simulink model "MJrlsfiltersystemidentification"  (R2023a)
settings: Solver=FixedStepDiscrete  StartTime=0.0  StopTime=Inf  RelTol=1e-3  EnableMultiTasking=on
PreLoadFcn:
  | Ts = 1/1e4;
  | L = 1024;
libraries: dspsrcs4 x2, dspsnks4 x1, dspmathops x1, dspadpt3 x1
CloseFcn:
  | clear Ts L
  | close all force
settings Model: Creator=The MathWorks, Inc.  LastModifiedBy=janssonm
settings SolverCC: AlgebraicLoopSolver=TrustRegion  MaxZcPerStep=1
settings DataIOCC: LimitDataPoints=on  SaveFormat=Array  ReturnWorkspaceOutputs=off
settings OptimizationCC: ReuseModelBlockBuffer=off  LifeSpan=inf  SimCompilerOptimization=on
settings DebuggingCC: UnderspecifiedInitializationDetection=Classic  MergeDetectMultiDrivingBlocksExec=none  SolverPrmCheckMsg=warning  UnconnectedInputMsg=warning  UnconnectedOutputMsg=warning  UnconnectedLineMsg=warning  AllowSymbolicDim=off  SFUnexpectedBacktrackingDiag=warning  SFNoUnconditionalDefaultTransitionDiag=warning  SFExecutionAtInitializationDiag=none  ArithmeticOperatorsInVariantConditions=warning
settings HardwareCC: ProdBitPerPointer=32  ProdBitPerSizeT=32  ProdBitPerPtrDiffT=32  ProdLargestAtomicFloat=None  ProdIntDivRoundTo=Undefined  ProdEndianess=Unspecified  ProdWordSize=32  ProdHWDeviceType=32-bit Generic
settings ModelReferenceCC: EnableRefExpFcnMdlSchedulingChecks=on  PropagateSignalLabelsOutOfModel=off
settings SFSimCC: SimUseLocalCustomCode=off  CustomCodeUndefinedFunction=UseInterfaceOnly
settings RTWCC: RTWUseLocalCustomCode=off  DLArmComputeVersion=19.05
settings CodeAppCC: StateflowObjectComments=on
settings GRTTargetCC: TargetLangStandard=C89/C90 (ANSI)
settings ConfigComp: CovMetricSettings=dw  CovSaveCumulativeToWorkspaceVar=on  CovSaveSingleToWorkspaceVar=on  CovExternalEMLEnable=off  CovSFcnEnable=off

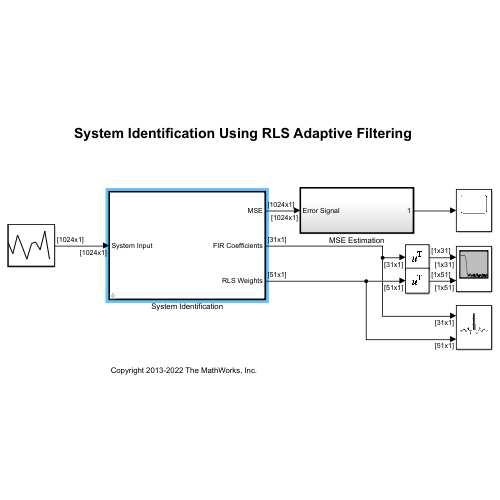
[thumbnail: Simulink's stored preview of the top-level diagram]
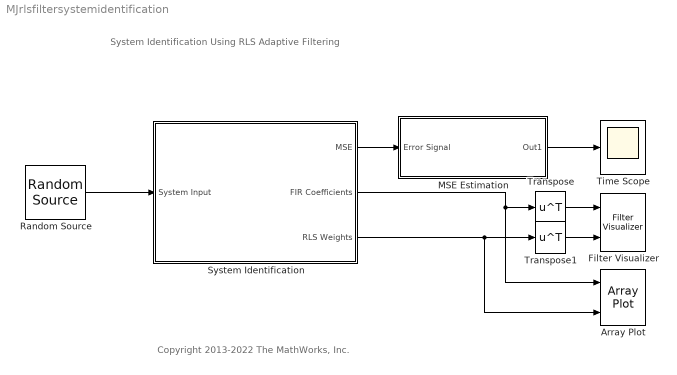
== system MJrlsfiltersystemidentification ==
  note: Copyright 2013-2022 The MathWorks, Inc.
  note: System Identification Using RLS Adaptive Filtering
  Array Plot : ArrayPlot  NumInputPorts=2  WindowPosition=[1528.000000,666.000000,363.000000,359.000000,]  Visible=on  ScopeFrameLocation=window  AxesScaling=Manual  Title=Desired and Estimated Filter coefficients  YLimits=[-0.2,1.2]  ShowLegend=on  DefaultConfigurationName=dsp.scopes.ArrayPlotBlockSpecification
  Filter Visualizer : dspsnks4/Filter Visualizer  NumFilters=2  FilterType=FIR  FFTLength=2048  NormalizedFrequency=off  SampleRate=44100  FrequencyRange=[0,22050]  XScale=Linear  MagnitudeDisplay=Magnitude (dB)  PlotAsMagnitudePhase=off  PlotType=Line  AxesScaling=Manual  AxesScalingNumUpdates=100  MaximizeAxes=Auto  Title=Magnitude Response  YLimits=[-80,20]  ShowLegend=on  FilterNames="[\"Unknow FIR System\",\"Estimated RLS System\"]"  ShowGrid=on  Visible=off  ExpandToolstrip=off
  MSE Estimation : Subsystem  TreatAsAtomicUnit=on
  Random Source : dspsrcs4/Random Source  SrcType=Gaussian  NormMethod=Ziggurat  CltLength=12  MinVal=0  MaxVal=1  MeanVal=0  VarVal=1e-2  RepMode=Specify seed  rawSeed=1  IsInherit=off  SampMode=Discrete  SampTime=Ts  SampFrame=L  DataType=Double  OutComplex=Real  OutputFrames=off
  System Identification : Subsystem  TreatAsAtomicUnit=on  mask{Fc=3.000e+03, lambda=0.999}
      mask prompts: Fc "Lowpass Filter Cutoff (Hz)"; lambda "RLS Forgetting Factor"
      mask DialogControl DescTextVar Prompt: System Identification Parameters
  Time Scope : Scope
  Transpose : Math  Operator=transpose
  Transpose1 : Math  Operator=transpose
  wires:
  Random Source/1 -> System Identification/1(System Input)
  System Identification/1(MSE) -> MSE Estimation/1(Error Signal)
  System Identification/2(FIR Coefficients) -> Transpose/1, Array Plot/1
  System Identification/3(RLS Weights) -> Transpose1/1, Array Plot/2
  Transpose/1 -> Filter Visualizer/1
  Transpose1/1 -> Filter Visualizer/2
  MSE Estimation/1(Out1) -> Time Scope/1

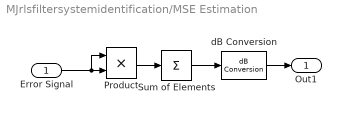
== system MJrlsfiltersystemidentification/MSE Estimation ==
  Error Signal : Inport
  Product : Product
  Sum of Elements : Sum  Inputs=+
  dB Conversion : dspmathops/dB Conversion  dBtype=dB  intype=Amplitude  R=1  fuzz=on
  Out1 : Outport
  wires:
  dB Conversion/1 -> Out1/1
  Error Signal/1 -> Product/1, Product/2
  Product/1 -> Sum of Elements/1
  Sum of Elements/1 -> dB Conversion/1

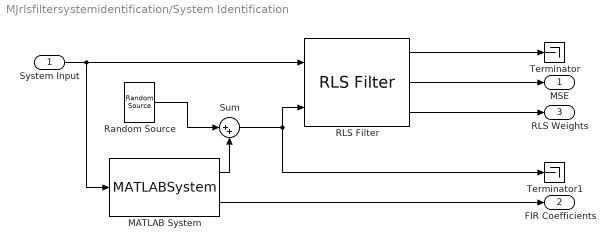
== system MJrlsfiltersystemidentification/System Identification ==
  System Input : Inport
  MATLAB System : MATLABSystem  System=VariableBandwidthFIRFilter  FilterOrder=30  FilterType=Lowpass  CutoffFrequencyPort=off  CutoffFrequency=Fc  CenterFrequencyPort=off  CenterFrequency=44100 / 4  BandwidthPort=off  Bandwidth=7680  Window=Hann  KaiserWindowParameter=.5  SidelobeAttenuation=60  SampleRateMode=Specify on dialog  SampleRate=44100  SimulateUsing=Interpreted execution
      mask Type: VariableBandwidthFIRFilter
      mask Display:
      | disp(['Variable' char(10) 'Bandwidth' char(10) 'FIR']);
      | port_label('output',1,'y');
      | port_label('output',2,'coeffs');
  RLS Filter : dspadpt3/RLS Filter  L=51  lambdaflag=Dialog  lambda=lambda  addnparflag=on  ic=0  delta=0.1  Adapt=off  resetflag=None  weights=on
  Random Source : dspsrcs4/Random Source  SrcType=Gaussian  NormMethod=Ziggurat  CltLength=12  MinVal=0  MaxVal=1  MeanVal=0  VarVal=1e-4  RepMode=Specify seed  rawSeed=11  IsInherit=off  SampMode=Discrete  SampTime=Ts  SampFrame=L  DataType=Single  OutComplex=Real  OutputFrames=off
  Sum : Sum  Inputs=|++
  Terminator : Terminator
  Terminator1 : Terminator
  MSE : Outport  VectorParamsAs1DForOutWhenUnconnected=off
  FIR Coefficients : Outport  Port=2  VectorParamsAs1DForOutWhenUnconnected=off
  RLS Weights : Outport  Port=3  VectorParamsAs1DForOutWhenUnconnected=off
  wires:
  System Input/1 -> RLS Filter/1, MATLAB System/1
  RLS Filter/1 -> Terminator/1
  RLS Filter/2 -> MSE/1
  MATLAB System/2 -> FIR Coefficients/1
  RLS Filter/3 -> RLS Weights/1
  Random Source/1 -> Sum/1
  MATLAB System/1 -> Sum/2
  Sum/1 -> Terminator1/1, RLS Filter/2
